simulink model "peopleTracker"  (R2020a)
settings: Solver=VariableStepAuto  StartTime=0.0  StopTime=10.0  RelTol=1e-3
settings Model: Creator=HannesDittmann  LastModifiedBy=HannesDittmann

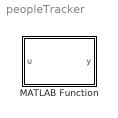
== system peopleTracker ==
  MATLAB Function : MATLAB Function  TreatAsAtomicUnit=on

== matlab function peopleTracker/MATLAB Function ==
  data: u input; y output
function y = fcn(u)

intrinsics2 = cameraIntrinsics([540.6860,479.750],[540.6860,269.7500],[540,960]);
sensor2 = monoCamera(intrinsics2,1.0,'Yaw',0);
d2.sensor = sensor2;

y = u;
